simulink model "opencircuit"  (Simulink 7.6)
settings: Solver=ode23tb  SolverMode=SingleTasking  StartTime=0.0  StopTime=0.2  RelTol=1e-4
libraries: powerlib x10
Description:
  | Copyright 2008-2010 The MathWorks, Inc.
settings Model: Creator=MathWorks  LastModifiedBy=ROOTS  ExtModeTrigMode=oneshot  ExtModeArmWhenConnect=off
settings DataIOCC: LimitDataPoints=off  SignalLoggingName=sigsOut
settings OptimizationCC: BooleanDataType=off  InlineInvariantSignals=on  InitFltsAndDblsToZero=on  EfficientMapNaN2IntZero=off
settings DebuggingCC: SaveWithParameterizedLinksMsg=none  SignalResolutionControl=TryResolveAllWithWarning  SolverPrmCheckMsg=none  MultiTaskDSMMsg=warning  MultiTaskCondExecSysMsg=none  SigSpecEnsureSampleTimeMsg=none  StrictBusMsg=None
settings HardwareCC: TargetUnknown=on
settings RTWCC: IncludeERTFirstTime=on
settings GRTTargetCC: TargetFcnLib=ansi_tfl_tmw.mat

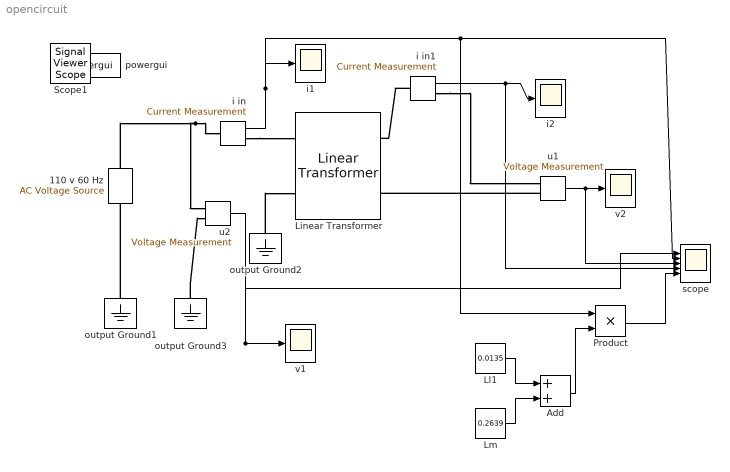
== system opencircuit ==
  110 v 60 Hz : powerlib/Electrical Sources/AC Voltage Source  Description=source block  DialogController=POWERSYS.PowerSysDialog  SystemSampleTime=-1  Amplitude=155.563  Phase=0  Frequency=60  SampleTime=0  Measurements=None
      settings: AttributesFormatString=\n
  Add : Sum
  Linear Transformer : powerlib/Elements/Linear Transformer  DialogController=POWERSYS.PowerSysDialog  PhysicalDomain=powersysdomain  SubClassName=unknown  LeftPortType=p1  RightPortType=p1  LConnTagsString=a|b  RConnTagsString=A|B  UNITS=SI  NominalPower=[75e3,60]  winding1=[110 6 0.0135]  winding2=[110 5 0.0135]  ThreeWindings=off  winding3=[120 0.00384 0]  RmLm=[99.5 0.2639]  Measurements=None  DataType=on
  Ll1 : Constant  Value=0.0135
  Lm : Constant  Value=0.2639
  Product : Product  RndMeth=Zero
  i in : powerlib/Measurements/Current Measurement  Tag=PoWeRsYsTeMmEaSuReMeNt  DialogController=POWERSYS.PowerSysDialog  SystemSampleTime=-1  PhasorSimulation=off  OutputType=Magnitude  PSBequivalent=0
  i in1 : powerlib/Measurements/Current Measurement  Tag=PoWeRsYsTeMmEaSuReMeNt  DialogController=POWERSYS.PowerSysDialog  SystemSampleTime=-1  PhasorSimulation=off  OutputType=Magnitude  PSBequivalent=0
  i1 : Scope
      settings: DeleteFcn=simscope BlockIsBeingDestroyed  PostSaveFcn=simscope Save  TickLabels=on  TimeRange=0.1  YMin=-10  YMax=10  SaveName=ScopeData3  DataFormat=Array
  i2 : Scope
      settings: DeleteFcn=simscope BlockIsBeingDestroyed  PostSaveFcn=simscope Save  TickLabels=on  TimeRange=0.1  YMin=-10  YMax=10  SaveName=ScopeData2  DataFormat=Array
  output Ground1 : powerlib/Elements/Ground  DialogController=POWERSYS.PowerSysDialog  PhysicalDomain=powersysdomain  SubClassName=unknown  LeftPortType=p1  RightPortType=p1  LConnTagsString=a
  output Ground2 : powerlib/Elements/Ground  DialogController=POWERSYS.PowerSysDialog  PhysicalDomain=powersysdomain  SubClassName=unknown  LeftPortType=p1  RightPortType=p1  LConnTagsString=a
  output Ground3 : powerlib/Elements/Ground  DialogController=POWERSYS.PowerSysDialog  PhysicalDomain=powersysdomain  SubClassName=unknown  LeftPortType=p1  RightPortType=p1  LConnTagsString=a
  powergui : powerlib/powergui  SystemSampleTime=-1  SimulationMode=Continuous  SampleTime=0  frequency=60  SPID=off  DisableSnubberDevices=off  DisableRonSwitches=off  DisableVfSwitches=off  SwTol=0  Interpol=off  frequencyindice=60  echomessages=off  HookPort=off  DisplayEquations=off  FunctionMessages=off  EnableUseOfTLC=off  x0status=blocks  RestoreLinks=warning  ResistiveCurrentMeasurement=off  Frange=[0:2:500]  Ylog=off  Xlog=on  ShowGrid=off  save=off  variable=ZData  ZoomFFT=on  StartTime=0.0  cycles=1  DisplayStyle=1  fundamental=60  FreqAxis=off  MaxFrequency=1000  frequencyindicesteady=1  RmsSteady=1  display=off  Ts=0  methode=off
  scope : Scope  NumInputPorts=5
      settings: DeleteFcn=simscope BlockIsBeingDestroyed  PostSaveFcn=simscope Save  TickLabels=on  TimeRange=0.2  YMin=-200~-5~-5~-5~-5  YMax=200~5~5~5~5  SaveName=ScopeData4  DataFormat=Array
  u1 : powerlib/Measurements/Voltage Measurement  Tag=PoWeRsYsTeMmEaSuReMeNt  DialogController=POWERSYS.PowerSysDialog  SystemSampleTime=-1  PhasorSimulation=off  OutputType=Magnitude  PSBequivalent=0
  u2 : powerlib/Measurements/Voltage Measurement  Tag=PoWeRsYsTeMmEaSuReMeNt  DialogController=POWERSYS.PowerSysDialog  SystemSampleTime=-1  PhasorSimulation=off  OutputType=Magnitude  PSBequivalent=0
  v1 : Scope
      settings: DeleteFcn=simscope BlockIsBeingDestroyed  PostSaveFcn=simscope Save  TickLabels=on  TimeRange=0.1  YMin=-200  YMax=200  DataFormat=Array
  v2 : Scope
      settings: DeleteFcn=simscope BlockIsBeingDestroyed  PostSaveFcn=simscope Save  TickLabels=on  TimeRange=0.1  YMin=-200  YMax=200  DataFormat=Array
  Scope1 : SignalViewerScope  IOType=viewer  RefreshTime=0.035000
  wires:
  i in/1 -> i1/1, scope/2, Product/1
  u2/1 -> v1/1, scope/1
  u1/1 -> v2/1, scope/3
  i in1/1 -> i2/1, scope/4
  Ll1/1 -> Add/1
  Lm/1 -> Add/2
  Add/1 -> Product/2
  Product/1 -> scope/5
  connections:
  output Ground1/LConn1 -- 110 v 60 Hz/LConn1
  110 v 60 Hz/RConn1 -- i in/LConn1 -- u2/LConn1
  output Ground3/LConn1 -- u2/LConn2
  i in1/RConn1 -- u1/LConn1
  u1/LConn2 -- Linear Transformer/RConn2
  i in1/LConn1 -- Linear Transformer/RConn1
  output Ground2/LConn1 -- Linear Transformer/LConn2
  i in/RConn1 -- Linear Transformer/LConn1
